simulink model "pid_control"  (R2020a)
settings: Solver=VariableStepAuto  StartTime=0.0  StopTime=10.0  RelTol=1e-3
settings Model: Creator=oyh  LastModifiedBy=oyh

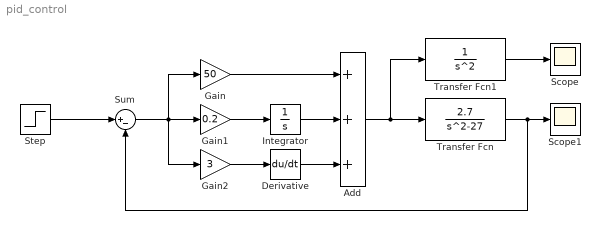
== system pid_control ==
  Add : Sum  Inputs=+++
  Derivative : Derivative
  Gain : Gain  Gain=50
  Gain1 : Gain  Gain=0.2
  Gain2 : Gain  Gain=3
  Integrator : Integrator
  Scope : Scope
  Scope1 : Scope
  Step : Step  SampleTime=0
  Sum : Sum  Inputs=|+-
  Transfer Fcn : TransferFcn  Numerator=[2.7]  Denominator=[1 0 -27]
  Transfer Fcn1 : TransferFcn  Denominator=[1 0 0]
  wires:
  Gain2/1 -> Derivative/1
  Gain1/1 -> Integrator/1
  Step/1 -> Sum/1
  Sum/1 -> Gain2/1, Gain1/1, Gain/1
  Add/1 -> Transfer Fcn1/1, Transfer Fcn/1
  Gain/1 -> Add/1
  Derivative/1 -> Add/3
  Integrator/1 -> Add/2
  Transfer Fcn/1 -> Sum/2, Scope1/1
  Transfer Fcn1/1 -> Scope/1
